simulink model "ShockCordSystem"  (R2022a)
settings: Solver=VariableStepAuto  StartTime=0.0  StopTime=5  RelTol=1e-5
model workspace (MAT data in the model file):
  CdSo_full = 13.9355
  K_m = 1
  K_s = 100
  Sig = Simulink.Signal
  Sig.DataType = 'auto'
  Sig.Dimensions = -1
  Sig.DimensionsMode = 'auto'
  Sig.Complexity = 'auto'
  Sig.SampleTime = -1
  Sig.SamplingMode = 'auto'
  ft_to_m = 0.3048
  g = 9.81
  m_x = 0.1
  m_y = 45
  tau_oe = 0.15
  tau_ol = 0.3
  v_desc = 112
settings Model: Creator=Artem Sotnikov  LastModifiedBy=Artem Sotnikov

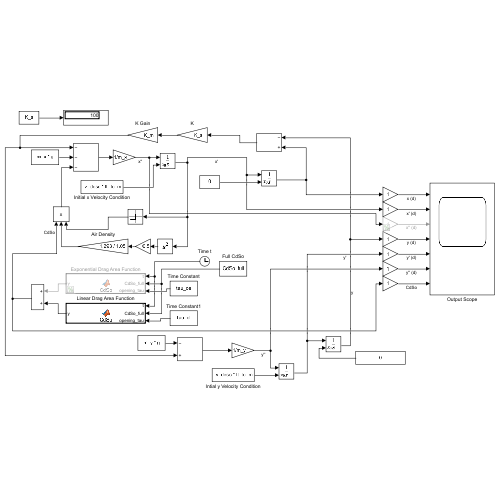
[thumbnail: Simulink's stored preview of the top-level diagram]
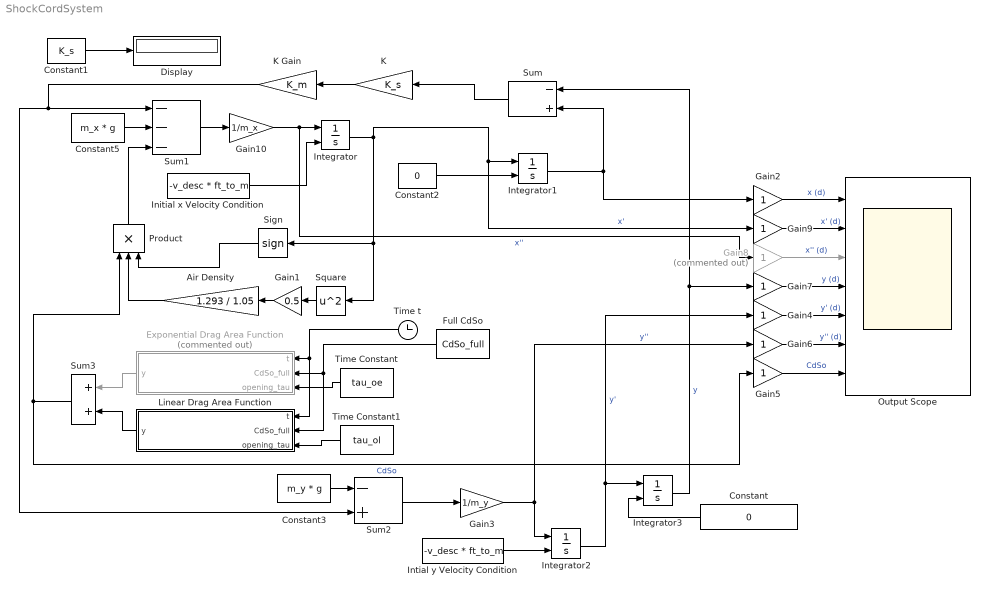
== system ShockCordSystem ==
  Air Density : Gain  Gain=1.293 / 1.05
  Constant : Constant  Value=0
  Constant1 : Constant  Value=K_s
  Constant2 : Constant  Value=0
  Constant3 : Constant  Value=m_y * g
  Constant5 : Constant  Value=m_x * g
  Display : Display
  Exponential Drag Area Function : MATLAB Function  Commented=on  TreatAsAtomicUnit=on
  Full CdSo : Constant  Value=CdSo_full
  Gain1 : Gain  Gain=0.5
  Gain10 : Gain  Gain=1/m_x
  Gain{2,4..7,9} (6 alike) : Gain
  Gain3 : Gain  Gain=1/m_y
  Gain8 : Gain  Commented=on
  Initial x Velocity Condition : Constant  Value=-v_desc * ft_to_m
  Integrator : Integrator  InitialConditionSource=external
  Integrator1 : Integrator  InitialConditionSource=external
  Integrator2 : Integrator  InitialConditionSource=external  InitialCondition=m_y * g
  Integrator3 : Integrator  InitialConditionSource=external
  Intial y Velocity Condition : Constant  Value=-v_desc * ft_to_m
  K : Gain  Gain=K_s
  K Gain : Gain  Gain=K_m
  Linear Drag Area Function : MATLAB Function  TreatAsAtomicUnit=on
  Output Scope : Scope  NumInputPorts=7
  Product : Product  Inputs=3
  Sign : Signum
  Square : Math  Operator=square
  Sum : Sum  Inputs=-+
  Sum1 : Sum  Inputs=---
  Sum2 : Sum  Inputs=-+
  Sum3 : Sum
  Time Constant : Constant  Value=tau_oe
  Time Constant1 : Constant  Value=tau_ol
  Time t : Clock
  wires:
  Integrator/1 -> Integrator1/1, Gain9/1, Sign/1, Square/1  "x'"
  Integrator2/1 -> Gain4/1, Integrator3/1  "y'"
  Sum/1 -> K/1
  Gain4/1 -> Output Scope/5  "y' (d)"
  Square/1 -> Gain1/1
  Product/1 -> Sum1/3
  Exponential Drag Area Function/1(y) -> Sum3/1
  Time t/1 -> Linear Drag Area Function/1(t), Exponential Drag Area Function/1(t)
  Gain1/1 -> Air Density/1
  Air Density/1 -> Product/2
  Sum2/1 -> Gain3/1
  K/1 -> K Gain/1
  Intial y Velocity Condition/1 -> Integrator2/2
  Initial x Velocity Condition/1 -> Integrator/2
  Constant/1 -> Integrator3/2
  Constant3/1 -> Sum2/1
  Constant5/1 -> Sum1/2
  Constant2/1 -> Integrator1/2
  Gain3/1 -> Integrator2/1, Gain6/1  "y''"
  Integrator3/1 -> Sum/1, Gain7/1  "y"
  Gain6/1 -> Output Scope/6  "y'' (d)"
  Gain7/1 -> Output Scope/4  "y (d)"
  Gain8/1 -> Output Scope/3  "x'' (d)"
  Gain9/1 -> Output Scope/2  "x' (d)"
  Gain2/1 -> Output Scope/1  "x (d)"
  Integrator1/1 -> Sum/2, Gain2/1
  Gain5/1 -> Output Scope/7  "CdSo"
  Sum1/1 -> Gain10/1
  Gain10/1 -> Gain8/1, Integrator/1  "x''"
  K Gain/1 -> Sum2/2, Sum1/1
  Time Constant/1 -> Exponential Drag Area Function/3(opening_tau)
  Sign/1 -> Product/3
  Sum3/1 -> Product/1, Gain5/1  "CdSo"
  Linear Drag Area Function/1(y) -> Sum3/2
  Time Constant1/1 -> Linear Drag Area Function/3(opening_tau)
  Full CdSo/1 -> Exponential Drag Area Function/2(CdSo_full), Linear Drag Area Function/2(CdSo_full)
  Constant1/1 -> Display/1

== matlab function ShockCordSystem/Linear Drag Area Function ==
  data: t input; CdSo_full input; opening_tau input; y output
function y  = CdSo(t, CdSo_full ...
    , opening_tau)


y = CdSo_full * (t / opening_tau);

if y > CdSo_full
    y = CdSo_full;
end

== matlab function ShockCordSystem/Exponential Drag Area Function ==
  data: y output; t input; CdSo_full input; opening_tau input
function y = CdSo(t, CdSo_full, opening_tau)

y = CdSo_full * (1 - exp(-t/opening_tau));
